simulink model "DSM_SIM"  (R2017b)
settings: Solver=FixedStepDiscrete  StartTime=0.0  StopTime=N/Fs  RelTol=1e-3
values from neighbouring files (symbols this model uses):
  ftest = 9e3    (= 9000)    [Model3.m]    (also in Model3_LTE.m = 2250)
  Ts = 1/Fs    (= 2.03450520833e-06)    [Model3.m]    (also in Model3_LTE.m = 1/Fs)
undefined symbols (not defined in the file or in its folder): a, b, c, g
libraries: dspsrcs4 x1
settings Model: Creator=o_cotte  LastModifiedBy=o_cotte

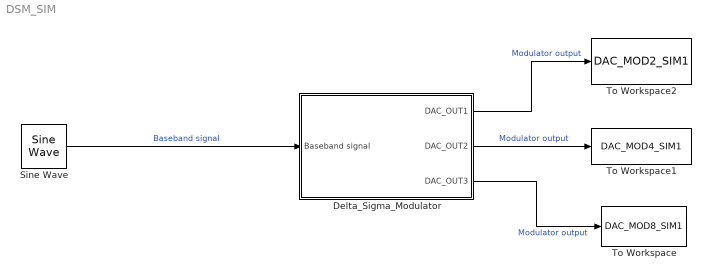
== system DSM_SIM ==
  Delta_Sigma_Modulator : Subsystem
  Sine Wave : dspsrcs4/Sine Wave  Amplitude=0.77  Frequency=ftest  Phase=0  SampleMode=Discrete  OutComplex=Real  CompMethod=Trigonometric fcn  TableSize=Speed  SampleTime=Ts  SamplesPerFrame=1  ResetState=Restart at time zero  OutputFrames=on  dataType=double  wordLen=16  udDataType=sfix(16)  fracBitsMode=Best precision  numFracBits=15  OutDataTypeStr=double  LastOutDataTypeStr=double
  To Workspace : ToWorkspace  VariableName=DAC_MOD8_SIM1  SampleTime=-1
  To Workspace1 : ToWorkspace  VariableName=DAC_MOD4_SIM1  SampleTime=-1
  To Workspace2 : ToWorkspace  VariableName=DAC_MOD2_SIM1  SampleTime=-1
  wires:
  Sine Wave/1 -> Delta_Sigma_Modulator/1(Baseband signal)  "Baseband signal"
  Delta_Sigma_Modulator/3(DAC_OUT3) -> To Workspace/1  "Modulator output"
  Delta_Sigma_Modulator/2(DAC_OUT2) -> To Workspace1/1  "Modulator output"
  Delta_Sigma_Modulator/1(DAC_OUT1) -> To Workspace2/1  "Modulator output"

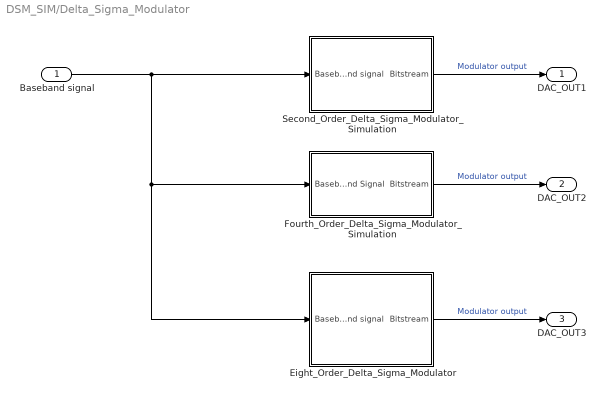
== system DSM_SIM/Delta_Sigma_Modulator ==
  Baseband signal : Inport
  Eight_Order_Delta_Sigma_Modulator : Subsystem
  Fourth_Order_Delta_Sigma_Modulator_Simulation : Subsystem
  Second_Order_Delta_Sigma_Modulator_Simulation : Subsystem
  DAC_OUT1 : Outport
  DAC_OUT2 : Outport  Port=2
  DAC_OUT3 : Outport  Port=3
  wires:
  Second_Order_Delta_Sigma_Modulator_Simulation/1(Bitstream) -> DAC_OUT1/1  "Modulator output"
  Fourth_Order_Delta_Sigma_Modulator_Simulation/1(Bitstream) -> DAC_OUT2/1  "Modulator output"
  Eight_Order_Delta_Sigma_Modulator/1(Bitstream) -> DAC_OUT3/1  "Modulator output"
  Baseband signal/1 -> Eight_Order_Delta_Sigma_Modulator/1(Baseband signal), Fourth_Order_Delta_Sigma_Modulator_Simulation/1(Baseband Signal), Second_Order_Delta_Sigma_Modulator_Simulation/1(Baseband signal)

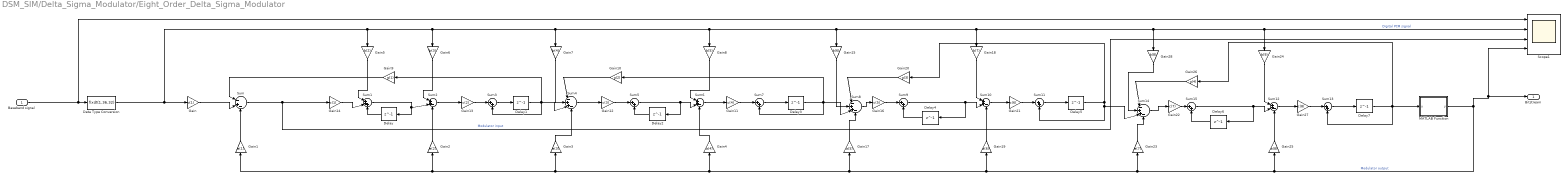
== system DSM_SIM/Delta_Sigma_Modulator/Eight_Order_Delta_Sigma_Modulator ==
  Baseband signal : Inport
  Data Type Conversion : DataTypeConversion  OutDataTypeStr=fixdt(1,36,32)
  Delay{,1..7} (8 alike) : Delay  DelayLength=1  InitialCondition=0
  Gain : Gain  Gain=b(1)  OutDataTypeStr=Inherit: Same as input  ParamDataTypeStr=Inherit: Same as input  LockScale=on
  Gain1 : Gain  Gain=a(1)  OutDataTypeStr=Inherit: Same as input
  Gain10 : Gain  Gain=g(2)  OutDataTypeStr=Inherit: Same as input  ParamDataTypeStr=Inherit: Same as input  LockScale=on
  Gain11 : Gain  Gain=c(4)  OutDataTypeStr=Inherit: Same as input  ParamDataTypeStr=Inherit: Same as input  LockScale=on
  Gain12 : Gain  Gain=c(3)  OutDataTypeStr=Inherit: Same as input  ParamDataTypeStr=Inherit: Same as input  LockScale=on
  Gain13 : Gain  Gain=c(2)  OutDataTypeStr=Inherit: Same as input  ParamDataTypeStr=Inherit: Same as input  LockScale=on
  Gain14 : Gain  Gain=c(1)  OutDataTypeStr=Inherit: Same as input  ParamDataTypeStr=Inherit: Same as input  LockScale=on
  Gain15 : Gain  Gain=b(6)  OutDataTypeStr=Inherit: Same as input  ParamDataTypeStr=Inherit: Same as input  LockScale=on
  Gain16 : Gain  Gain=c(5)  OutDataTypeStr=Inherit: Same as input  ParamDataTypeStr=Inherit: Same as input  LockScale=on
  Gain17 : Gain  Gain=a(5)  OutDataTypeStr=Inherit: Same as input
  Gain18 : Gain  Gain=b(7)  OutDataTypeStr=Inherit: Same as input  ParamDataTypeStr=Inherit: Same as input  LockScale=on
  Gain19 : Gain  Gain=a(6)  OutDataTypeStr=Inherit: Same as input
  Gain2 : Gain  Gain=a(2)  OutDataTypeStr=Inherit: Same as input
  Gain20 : Gain  Gain=g(3)  OutDataTypeStr=Inherit: Same as input  ParamDataTypeStr=Inherit: Same as input  LockScale=on
  Gain21 : Gain  Gain=c(6)  OutDataTypeStr=Inherit: Same as input  ParamDataTypeStr=Inherit: Same as input  LockScale=on
  Gain22 : Gain  Gain=c(7)  OutDataTypeStr=Inherit: Same as input  ParamDataTypeStr=Inherit: Same as input  LockScale=on
  Gain23 : Gain  Gain=a(7)  OutDataTypeStr=Inherit: Same as input
  Gain24 : Gain  Gain=b(9)  OutDataTypeStr=Inherit: Same as input  ParamDataTypeStr=Inherit: Same as input  LockScale=on
  Gain25 : Gain  Gain=a(8)  OutDataTypeStr=Inherit: Same as input
  Gain26 : Gain  Gain=g(4)  OutDataTypeStr=Inherit: Same as input  ParamDataTypeStr=Inherit: Same as input  LockScale=on
  Gain27 : Gain  Gain=c(8)  OutDataTypeStr=Inherit: Same as input  ParamDataTypeStr=Inherit: Same as input  LockScale=on
  Gain28 : Gain  Gain=b(8)  OutDataTypeStr=Inherit: Same as input  ParamDataTypeStr=Inherit: Same as input  LockScale=on
  Gain3 : Gain  Gain=a(3)  OutDataTypeStr=Inherit: Same as input
  Gain4 : Gain  Gain=a(4)  OutDataTypeStr=Inherit: Same as input
  Gain5 : Gain  Gain=b(2)  OutDataTypeStr=Inherit: Same as input  ParamDataTypeStr=Inherit: Same as input  LockScale=on
  Gain6 : Gain  Gain=b(3)  OutDataTypeStr=Inherit: Same as input  ParamDataTypeStr=Inherit: Same as input  LockScale=on
  Gain7 : Gain  Gain=b(4)  OutDataTypeStr=Inherit: Same as input  ParamDataTypeStr=Inherit: Same as input  LockScale=on
  Gain8 : Gain  Gain=b(5)  OutDataTypeStr=Inherit: Same as input  ParamDataTypeStr=Inherit: Same as input  LockScale=on
  Gain9 : Gain  Gain=g(1)  OutDataTypeStr=Inherit: Same as input  ParamDataTypeStr=Inherit: Same as input  LockScale=on
  MATLAB Function : MATLAB Function  TreatAsAtomicUnit=on
  Scope1 : Scope  NumInputPorts=4
  Sum : Sum  Inputs=|-+-  OutDataTypeStr=Inherit: Same as accumulator  LockScale=on
  Sum1 : Sum  Inputs=|+++  OutDataTypeStr=Inherit: Same as accumulator  LockScale=on
  Sum{2,6,10,12} (4 alike) : Sum  Inputs=|++-  OutDataTypeStr=Inherit: Same as accumulator  LockScale=on
  Sum{3,5,7,9,11,13,15} (7 alike) : Sum  Inputs=|++  OutDataTypeStr=Inherit: Same as accumulator  LockScale=on
  Sum14 : Sum  Inputs=|-++-  OutDataTypeStr=Inherit: Same as accumulator  LockScale=on
  Sum4 : Sum  Inputs=|-++-  OutDataTypeStr=Inherit: Same as accumulator  LockScale=on
  Sum8 : Sum  Inputs=|-++-  OutDataTypeStr=Inherit: Same as accumulator  LockScale=on
  Bitstream : Outport
  wires:
  Delay5/1 -> Sum14/3, Sum11/2, Gain20/1
  Gain27/1 -> Sum13/1
  Gain26/1 -> Sum14/1
  Gain16/1 -> Sum9/1
  Gain13/1 -> Sum3/1
  Gain6/1 -> Sum2/1
  Delay7/1 -> MATLAB Function/1(u), Sum13/2, Gain26/1
  Gain7/1 -> Sum4/2
  Gain23/1 -> Sum14/4
  Gain28/1 -> Sum14/2
  Gain19/1 -> Sum10/3
  Gain24/1 -> Sum12/1
  Delay4/1 -> Sum9/2
  Gain15/1 -> Sum8/2
  Sum15/1 -> Delay6/1, Sum12/2
  Gain22/1 -> Sum15/1
  Gain25/1 -> Sum12/3
  Sum13/1 -> Delay7/1
  Sum14/1 -> Gain22/1
  Gain18/1 -> Sum10/1
  MATLAB Function/1(y) -> Bitstream/1, Scope1/4, Gain25/1, Gain23/1, Gain19/1, Gain17/1, Gain1/1, Gain2/1, Gain3/1, Gain4/1  "Modulator output"
  Sum8/1 -> Gain16/1
  Delay6/1 -> Sum15/2
  Sum5/1 -> Delay2/1, Sum6/2
  Baseband signal/1 -> Data Type Conversion/1, Scope1/1
  Gain14/1 -> Sum1/2
  Sum6/1 -> Gain11/1
  Data Type Conversion/1 -> Gain5/1, Gain8/1, Gain18/1, Gain28/1, Gain24/1, Scope1/2, Gain15/1, Gain7/1, Gain6/1, Gain/1  "Digital PCM signal"
  Sum12/1 -> Gain27/1
  Sum/1 -> Scope1/3, Gain14/1  "Modulator input"
  Delay2/1 -> Sum5/2
  Delay1/1 -> Sum3/2, Gain9/1, Sum4/3
  Sum9/1 -> Delay4/1, Sum10/2
  Sum4/1 -> Gain12/1
  Sum11/1 -> Delay5/1
  Sum2/1 -> Gain13/1
  Gain20/1 -> Sum8/1
  Sum7/1 -> Delay3/1
  Gain5/1 -> Sum1/1
  Gain8/1 -> Sum6/1
  Gain10/1 -> Sum4/1
  Gain11/1 -> Sum7/1
  Gain21/1 -> Sum11/1
  Gain/1 -> Sum/2
  Sum1/1 -> Delay/1, Sum2/2
  Gain12/1 -> Sum5/1
  Gain9/1 -> Sum/1
  Gain4/1 -> Sum6/3
  Gain17/1 -> Sum8/4
  Sum10/1 -> Gain21/1
  Delay3/1 -> Sum8/3, Sum7/2, Gain10/1
  Gain2/1 -> Sum2/3
  Gain3/1 -> Sum4/4
  Gain1/1 -> Sum/3
  Delay/1 -> Sum1/3
  Sum3/1 -> Delay1/1

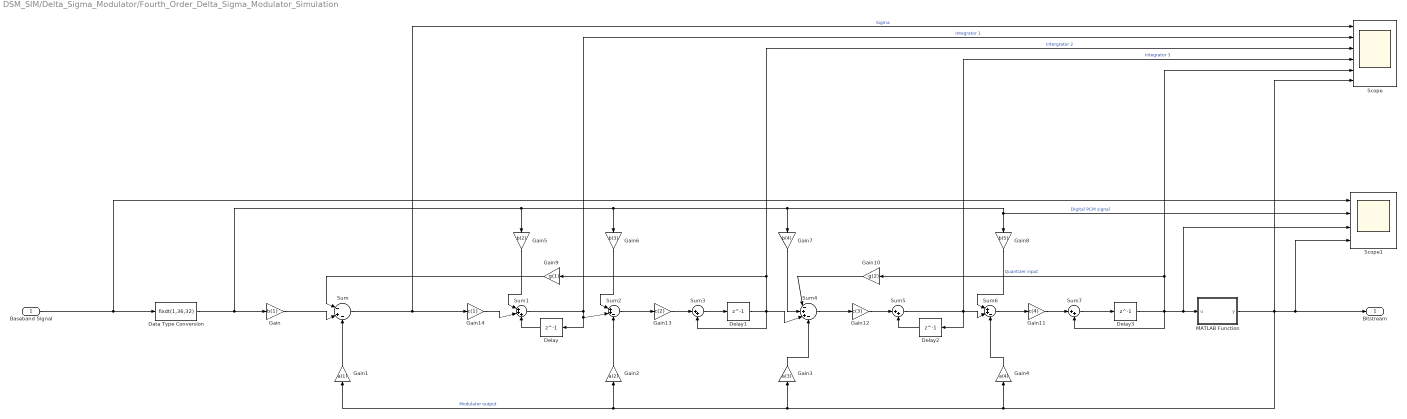
== system DSM_SIM/Delta_Sigma_Modulator/Fourth_Order_Delta_Sigma_Modulator_Simulation ==
  Baseband Signal : Inport
  Data Type Conversion : DataTypeConversion  OutDataTypeStr=fixdt(1,36,32)
  Delay{,1..3} (4 alike) : Delay  DelayLength=1  InitialCondition=0
  Gain : Gain  Gain=b(1)  OutDataTypeStr=Inherit: Same as input  ParamDataTypeStr=Inherit: Same as input  LockScale=on
  Gain1 : Gain  Gain=a(1)  OutDataTypeStr=Inherit: Same as input
  Gain10 : Gain  Gain=g(2)  OutDataTypeStr=Inherit: Same as input  ParamDataTypeStr=Inherit: Same as input  LockScale=on
  Gain11 : Gain  Gain=c(4)  OutDataTypeStr=Inherit: Same as input  ParamDataTypeStr=Inherit: Same as input  LockScale=on
  Gain12 : Gain  Gain=c(3)  OutDataTypeStr=Inherit: Same as input  ParamDataTypeStr=Inherit: Same as input  LockScale=on
  Gain13 : Gain  Gain=c(2)  OutDataTypeStr=Inherit: Same as input  ParamDataTypeStr=Inherit: Same as input  LockScale=on
  Gain14 : Gain  Gain=c(1)  OutDataTypeStr=Inherit: Same as input  ParamDataTypeStr=Inherit: Same as input  LockScale=on
  Gain2 : Gain  Gain=a(2)  OutDataTypeStr=Inherit: Same as input
  Gain3 : Gain  Gain=a(3)  OutDataTypeStr=Inherit: Same as input
  Gain4 : Gain  Gain=a(4)  OutDataTypeStr=Inherit: Same as input
  Gain5 : Gain  Gain=b(2)  OutDataTypeStr=Inherit: Same as input  ParamDataTypeStr=Inherit: Same as input  LockScale=on
  Gain6 : Gain  Gain=b(3)  OutDataTypeStr=Inherit: Same as input  ParamDataTypeStr=Inherit: Same as input  LockScale=on
  Gain7 : Gain  Gain=b(4)  OutDataTypeStr=Inherit: Same as input  ParamDataTypeStr=Inherit: Same as input  LockScale=on
  Gain8 : Gain  Gain=b(5)  OutDataTypeStr=Inherit: Same as input  ParamDataTypeStr=Inherit: Same as input  LockScale=on
  Gain9 : Gain  Gain=g(1)  OutDataTypeStr=Inherit: Same as input  ParamDataTypeStr=Inherit: Same as input  LockScale=on
  MATLAB Function : MATLAB Function  TreatAsAtomicUnit=on
  Scope : Scope  NumInputPorts=6
  Scope1 : Scope  NumInputPorts=4
  Sum : Sum  Inputs=|-+-  OutDataTypeStr=Inherit: Same as accumulator  LockScale=on
  Sum1 : Sum  Inputs=|+++  OutDataTypeStr=Inherit: Same as accumulator  LockScale=on
  Sum2 : Sum  Inputs=|++-  OutDataTypeStr=Inherit: Same as accumulator  LockScale=on
  Sum3 : Sum  Inputs=|++  OutDataTypeStr=Inherit: Same as accumulator  LockScale=on
  Sum4 : Sum  Inputs=|-++-  OutDataTypeStr=Inherit: Same as accumulator  LockScale=on
  Sum5 : Sum  Inputs=|++  OutDataTypeStr=Inherit: Same as accumulator  LockScale=on
  Sum6 : Sum  Inputs=|++-  OutDataTypeStr=Inherit: Same as accumulator  LockScale=on
  Sum7 : Sum  Inputs=|++  OutDataTypeStr=Inherit: Same as accumulator  LockScale=on
  Bitstream : Outport
  wires:
  Sum1/1 -> Scope/2, Delay/1, Sum2/2  "Integrator 1"
  Sum3/1 -> Delay1/1
  Gain5/1 -> Sum1/1
  Delay3/1 -> Scope1/3, MATLAB Function/1(u), Sum7/2, Scope/5, Gain10/1  "Quantizer input"
  MATLAB Function/1(y) -> Scope/6, Bitstream/1, Scope1/4, Gain1/1, Gain2/1, Gain3/1, Gain4/1  "Modulator output"
  Sum4/1 -> Gain12/1
  Gain11/1 -> Sum7/1
  Sum2/1 -> Gain13/1
  Gain6/1 -> Sum2/1
  Gain7/1 -> Sum4/2
  Gain10/1 -> Sum4/1
  Gain13/1 -> Sum3/1
  Sum5/1 -> Scope/4, Delay2/1, Sum6/2  "Integrator 3"
  Gain/1 -> Sum/2
  Baseband Signal/1 -> Data Type Conversion/1, Scope1/1
  Delay2/1 -> Sum5/2
  Data Type Conversion/1 -> Gain5/1, Gain8/1, Scope1/2, Gain7/1, Gain6/1, Gain/1  "Digital PCM signal"
  Sum6/1 -> Gain11/1
  Gain2/1 -> Sum2/3
  Gain8/1 -> Sum6/1
  Gain14/1 -> Sum1/2
  Gain3/1 -> Sum4/4
  Gain4/1 -> Sum6/3
  Delay/1 -> Sum1/3
  Sum7/1 -> Delay3/1
  Gain12/1 -> Sum5/1
  Gain1/1 -> Sum/3
  Gain9/1 -> Sum/1
  Sum/1 -> Scope/1, Gain14/1  "Sigma"
  Delay1/1 -> Sum3/2, Scope/3, Gain9/1, Sum4/3  "Intergrator 2"

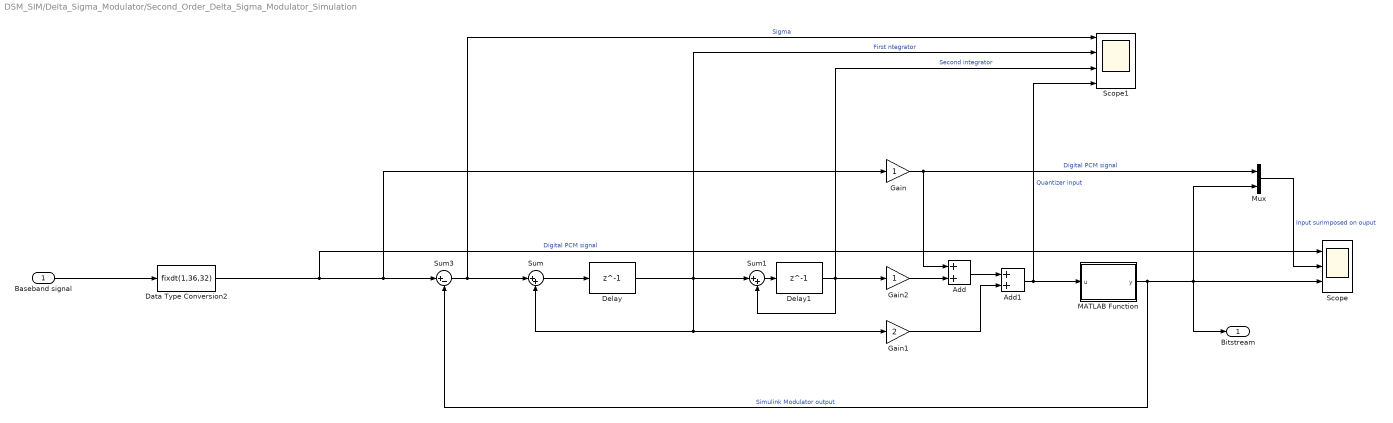
== system DSM_SIM/Delta_Sigma_Modulator/Second_Order_Delta_Sigma_Modulator_Simulation ==
  Baseband signal : Inport
  Add : Sum  OutDataTypeStr=Inherit: Same as accumulator  LockScale=on
  Add1 : Sum  OutDataTypeStr=Inherit: Same as accumulator
  Data Type Conversion2 : DataTypeConversion  OutDataTypeStr=fixdt(1,36,32)  LockScale=on
  Delay : Delay  DelayLength=1  InitialCondition=0  InputProcessing=Columns as channels (frame based)
  Delay1 : Delay  DelayLength=1  InitialCondition=0  InputProcessing=Columns as channels (frame based)
  Gain : Gain  OutDataTypeStr=Inherit: Same as input  LockScale=on
  Gain1 : Gain  Gain=2  OutDataTypeStr=Inherit: Same as input  ParamDataTypeStr=Inherit: Same as input  LockScale=on
  Gain2 : Gain  OutDataTypeStr=Inherit: Same as input  LockScale=on
  MATLAB Function : MATLAB Function  TreatAsAtomicUnit=on
  Mux : Mux  Inputs=2
  Scope : Scope  NumInputPorts=3
  Scope1 : Scope  NumInputPorts=4
  Sum : Sum  Inputs=|++  OutDataTypeStr=Inherit: Same as accumulator
  Sum1 : Sum  Inputs=|++  OutDataTypeStr=Inherit: Same as accumulator
  Sum3 : Sum  Inputs=|+-  OutDataTypeStr=Inherit: Same as accumulator
  Bitstream : Outport
  wires:
  Mux/1 -> Scope/2  "Input surimposed on ouput"
  Gain2/1 -> Add/2
  Sum/1 -> Delay/1
  Gain1/1 -> Add1/2
  Delay1/1 -> Gain2/1, Scope1/3, Sum1/2  "Second integrator"
  Sum1/1 -> Delay1/1
  MATLAB Function/1(y) -> Sum3/2, Bitstream/1, Mux/2, Scope/3  "Simulink Modulator output"
  Delay/1 -> Scope1/2, Sum1/1, Gain1/1, Sum/2  "First ntegrator"
  Gain/1 -> Add/1, Mux/1  "Digital PCM signal"
  Sum3/1 -> Sum/1, Scope1/1  "Sigma"
  Data Type Conversion2/1 -> Gain/1, Sum3/1, Scope/1  "Digital PCM signal"
  Add/1 -> Add1/1
  Baseband signal/1 -> Data Type Conversion2/1
  Add1/1 -> MATLAB Function/1(u), Scope1/4  "Quantizer input"

== matlab function DSM_SIM/Delta_Sigma_Modulator/Second_Order_Delta_Sigma_Modulator_Simulation/MATLAB Function ==
  data: u input; y output
function y = fcn(u)
%#codegen
% nLev=2;
% st=fi(nLev-2,1,36,30);
% y=fi(0,1,36,30);
% if u < -st
%     y = fi(-nLev+1,1,36,30);
% elseif u >= st
%     y = fi(nLev-1,1,36,30);
% else
%     for n=1:nLev-2
%         k=fi(n,1,36,30);
%         if u >= -nLev + 2*k && u < -nLev + 2*(k+1)
%             y = fi(2*k-1-nLev,1,36,30);
%         end
%     end
% end
% nLev=64;
% st=fi(nLev-2,1,36,25);
% y=fi(0,1,36,25);
% for n=1:nLev-2
%     k=fi(n,1,36,25);
%     if u < -st
%         y = fi(-nLev+1,1,36,25);
%         break;
%     elseif u >= st
%         y = fi(nLev-1,1,36,25);
%         break;
%     elseif u >= -nLev + 2*k && u < -nLev + 2*(k+1)
%         y = fi(2*k-1-nLev,1,36,25);
%         break;
%     end
% end

if u < 0
    y = fi(-1,1,36,32);
    %y = -1;
else
    y = fi(1,1,36,32);
    %y = 1;
end

% if u < -14
%     y = fi(-15,1,36,28);
% elseif u >= -14 && u < -12
%     y = fi(-13,1,36,28);
% elseif u >= -12 && u < -10
%     y = fi(-11,1,36,28);
% elseif u >= -10 && u < -8
%     y = fi(-9,1,36,28);
% elseif u >= -8 && u < -6
%     y = fi(-7,1,36,28);
% elseif u >= -6 && u < -4
%     y = fi(-5,1,36,28);
% elseif u >= -4 && u < -2
%     y = fi(-3,1,36,28);
% elseif u >= -2 && u < 0
%     y = fi(-1,1,36,28);
% elseif u >= 0 && u < 2
%     y = fi(1,1,36,28);
% elseif u >= 2 && u < 4
%     y = fi(3,1,36,28);
% elseif u >= 4 && u < 6
%     y = fi(5,1,36,28);
% elseif u >= 6 && u < 8
%     y = fi(7,1,36,28);
% elseif u >= 8 && u < 10
%     y = fi(9,1,36,28);
% elseif u >= 10 && u < 12
%     y = fi(11,1,36,28);
% elseif u >= 12 && u < 14
%     y = fi(13,1,36,28);
% else % u > 14
%     y = fi(15,1,36,28);
% end

== matlab function DSM_SIM/Delta_Sigma_Modulator/Fourth_Order_Delta_Sigma_Modulator_Simulation/MATLAB Function ==
  data: u input; y output
function y = fcn(u)
%#codegen
% nLev=64;
% st=fi(nLev-2,1,36,28);
% y=fi(1,1,36,28);
% for n=1:nLev-2
%     k=fi(n,1,36,28);
%     if u < -st
%         y=fi(-nLev+1,1,36,28);
%         break;
%     elseif u > st
%         y=fi(nLev-1,1,36,28);
%         break;
%     elseif u >= -nLev + 2*k && u <= -nLev + 2*(k+1)
%         y=fi(2*k-1-nLev,1,36,28);
%         break;
%     end
% end

% 2-level
if u < 0
    y = fi(-1,1,36,32);
    %y = -1;
else
    y = fi(1,1,36,32);
    %y = 1;
end

% 4-level
% if u < -2
%     y = fi(-3,1,36,28);
% elseif u > -2 && u < 0
%     y = fi(-1,1,36,28);
% elseif u >= 0 && u < 2
%     y = fi(1,1,36,28);
% else
%     y = fi(3,1,36,28);
% end

% 64-level
% if u < -62
%     y = fi(-63,1,36,28);
% elseif u >= -62 && u < -60
%     y = fi(-61,1,36,28);
% elseif u >= -60 && u < -58
%     y = fi(-59,1,36,28);
% elseif u >= -58 && u < -56
%     y = fi(-57,1,36,28);
% elseif u >= -56 && u < -54
%     y = fi(-55,1,36,28);
% elseif u >= -54 && u < -52
%     y = fi(-53,1,36,28);
% elseif u >= -52 && u < -50
%     y = fi(-51,1,36,28);
% elseif u >= -50 && u < -48
%     y = fi(-49,1,36,28);
% elseif u >= -48 && u < -46
%     y = fi(-47,1,36,28);
% elseif u >= -46 && u < -44
%     y = fi(-45,1,36,28);
% elseif u >= -44 && u < -42
%     y = fi(-43,1,36,28);
% elseif u >= -42 && u < -40
%     y = fi(-41,1,36,28);
% elseif u >= -40 && u < -38
%     y = fi(-39,1,36,28);
% elseif u >= -38 && u < -36
%     y = fi(-37,1,36,28);
% elseif u >= -36 && u < -34
%     y = fi(-35,1,36,28);
% elseif u >= -34 && u < -32
%     y = fi(-33,1,36,28);
% elseif u >= -32 && u < -30
%     y = fi(-31,1,36,28);
% elseif u >= -30 && u < -28
%     y = fi(-29,1,36,28);
% elseif u >= -28 && u < -26
%     y = fi(-27,1,36,28);
% elseif u >= -26 && u < -24
%     y = fi(-25,1,36,28);
% elseif u >= -24 && u < -22
%     y = fi(-23,1,36,28);
% elseif u >= -22 && u < -20
%     y = fi(-21,1,36,28);
% elseif u >= -20 && u < -18
%     y = fi(-19,1,36,28);
% elseif u >= -18 && u < -16
%     y = fi(-17,1,36,28);
% elseif u >= -16 && u < -14
%     y = fi(-15,1,36,28);
% elseif u >= -14 && u < -12
%     y = fi(-13,1,36,28);
% elseif u >= -12 && u < -10
%     y = fi(-11,1,36,28);
% elseif u >= -10 && u < -8
%     y = fi(-9,1,36,28);
% elseif u >= -8 && u < -6
%     y = fi(-7,1,36,28);
% elseif u >= -6 && u < -4
%     y = fi(-5,1,36,28);
% elseif u >= -4 && u < -2
%     y = fi(-3,1,36,28);
% elseif u >= -2 && u < 0
%     y = fi(-1,1,36,28);
% elseif u >= 0 && u < 2
%     y = fi(1,1,36,28);
% elseif u >= 2 && u < 4
%     y = fi(3,1,36,28);
% elseif u >= 4 && u < 6
%     y = fi(5,1,36,28);
% elseif u >= 6 && u < 8
%     y = fi(7,1,36,28);
% elseif u >= 8 && u < 10
%     y = fi(9,1,36,28);
% elseif u >= 10 && u < 12
%     y = fi(11,1,36,28);
% elseif u >= 12 && u < 14
%     y = fi(13,1,36,28);
% elseif u >= 14 && u < 16
%     y = fi(15,1,36,28);
% elseif u >= 16 && u < 18
%     y = fi(17,1,36,28);
% elseif u >= 18 && u < 20
%     y = fi(19,1,36,28);
% elseif u >= 20 && u < 22
%     y = fi(21,1,36,28);
% elseif u >= 22 && u < 24
%     y = fi(23,1,36,28);
% elseif u >= 24 && u < 26
%     y = fi(25,1,36,28);
% elseif u >= 26 && u < 28
%     y = fi(27,1,36,28);
% elseif u >= 28 && u < 30
%     y = fi(29,1,36,28);
% elseif u >= 30 && u < 32
%     y = fi(31,1,36,28);
% elseif u >= 32 && u < 34
%     y = fi(33,1,36,28);
% elseif u >= 34 && u < 36
%     y = fi(35,1,36,28);
% elseif u >= 36 && u < 38
%     y = fi(37,1,36,28);
% elseif u >= 38 && u < 40
%     y = fi(39,1,36,28);
% elseif u >= 40 && u < 42
%     y = fi(41,1,36,28);
% elseif u >= 42 && u < 44
%     y = fi(43,1,36,28);
% elseif u >= 44 && u < 46
%     y = fi(45,1,36,28);
% elseif u >= 46 && u < 48
%     y = fi(47,1,36,28);
% elseif u >= 48 && u < 50
%     y = fi(49,1,36,28);
% elseif u >= 50 && u < 52
%     y = fi(51,1,36,28);
% elseif u >= 52 && u < 54
%     y = fi(53,1,36,28);
% elseif u >= 54 && u < 56
%     y = fi(55,1,36,28);
% elseif u >= 56 && u < 58
%     y = fi(57,1,36,28);
% elseif u >= 58 && u < 60
%     y = fi(59,1,36,28);
% elseif u >= 60 && u < 62
%     y = fi(61,1,36,28);
% else % u > 62
%     y = fi(63,1,36,28);
% end

% 32-level
% if u < -30
%     y = fi(-31,1,36,28);
% elseif u >= -30 && u < -28
%     y = fi(-29,1,36,28);
% elseif u >= -28 && u < -26
%     y = fi(-27,1,36,28);
% elseif u >= -26 && u < -24
%     y = fi(-25,1,36,28);
% elseif u >= -24 && u < -22
%     y = fi(-23,1,36,28);
% elseif u >= -22 && u < -20
%     y = fi(-21,1,36,28);
% elseif u >= -20 && u < -18
%     y = fi(-19,1,36,28);
% elseif u >= -18 && u < -16
%     y = fi(-17,1,36,28);
% elseif u >= -16 && u < -14
%     y = fi(-15,1,36,28);
% elseif u >= -14 && u < -12
%     y = fi(-13,1,36,28);
% elseif u >= -12 && u < -10
%     y = fi(-11,1,36,28);
% elseif u >= -10 && u < -8
%     y = fi(-9,1,36,28);
% elseif u >= -8 && u < -6
%     y = fi(-7,1,36,28);
% elseif u >= -6 && u < -4
%     y = fi(-5,1,36,28);
% elseif u >= -4 && u < -2
%     y = fi(-3,1,36,28);
% elseif u >= -2 && u < 0
%     y = fi(-1,1,36,28);
% elseif u >= 0 && u < 2
%     y = fi(1,1,36,28);
% elseif u >= 2 && u < 4
%     y = fi(3,1,36,28);
% elseif u >= 4 && u < 6
%     y = fi(5,1,36,28);
% elseif u >= 6 && u < 8
%     y = fi(7,1,36,28);
% elseif u >= 8 && u < 10
%     y = fi(9,1,36,28);
% elseif u >= 10 && u < 12
%     y = fi(11,1,36,28);
% elseif u >= 12 && u < 14
%     y = fi(13,1,36,28);
% elseif u >= 14 && u < 16
%     y = fi(15,1,36,28);
% elseif u >= 16 && u < 18
%     y = fi(17,1,36,28);
% elseif u >= 18 && u < 20
%     y = fi(19,1,36,28);
% elseif u >= 20 && u < 22
%     y = fi(21,1,36,28);
% elseif u >= 22 && u < 24
%     y = fi(23,1,36,28);
% elseif u >= 24 && u < 26
%     y = fi(25,1,36,28);
% elseif u >= 26 && u < 28
%     y = fi(27,1,36,28);
% elseif u >= 28 && u < 30
%     y = fi(29,1,36,28);
% else % u > 30
%     y = fi(31,1,36,28);
% end

== matlab function DSM_SIM/Delta_Sigma_Modulator/Eight_Order_Delta_Sigma_Modulator/MATLAB Function ==
  data: u input; y output
function y = fcn(u)
%#codegen
% nLev=32;
% st=fi(nLev-2,1,36,28);
% y=fi(1,1,36,28);
% for n=1:nLev-2
%     k=fi(n,1,36,28);
%     if u < -st
%         y=fi(-nLev+1,1,36,28);
%         break;
%     elseif u > st
%         y=fi(nLev-1,1,36,28);
%         break;
%     elseif u >= -nLev + 2*k && u <= -nLev + 2*(k+1)
%         y=fi(2*k-1-nLev,1,36,28);
%         break;
%     end
% end
% nLev=2;
% st=fi(nLev,1,36,28);
% y=fi(0,1,36,28);
% for n=1:nLev
%     k=fi(n,1,36,28);
%     if u < -st+2
%         y = fi(-nLev+1,1,36,28);
%         break;
%     elseif u < -nLev + 2*k && u > -nLev + 2*(k+1)
%         y = fi(-nLev+1,1,36,28);
%         break;
%     elseif u >= nLev - 2*k && u < nLev - 2*(k+1)
%         y = fi(-nLev+1,1,36,28);
%         break;
%     else u > st-2
%         y = fi(nLev-1,1,36,28);
%         break;
%     end
% end

% 2-level
% if u < 0
%     y = -1;
% else
%     y = 1;
% end

% 2-level
if u < 0
    y = fi(-1,1,36,32);
else
    y = fi(1,1,36,32);
end

% 4-level
% if u < -2
%     y = fi(-3,1,36,28);
% elseif u > -2 && u < 0
%     y = fi(-1,1,36,28);
% elseif u >= 0 && u < 2
%     y = fi(1,1,36,28);
% else
%     y = fi(3,1,36,28);
% end

% 64-level
% if u < -62
%     y = fi(-63,1,36,28);
% elseif u >= -62 && u < -60
%     y = fi(-61,1,36,28);
% elseif u >= -60 && u < -58
%     y = fi(-59,1,36,28);
% elseif u >= -58 && u < -56
%     y = fi(-57,1,36,28);
% elseif u >= -56 && u < -54
%     y = fi(-55,1,36,28);
% elseif u >= -54 && u < -52
%     y = fi(-53,1,36,28);
% elseif u >= -52 && u < -50
%     y = fi(-51,1,36,28);
% elseif u >= -50 && u < -48
%     y = fi(-49,1,36,28);
% elseif u >= -48 && u < -46
%     y = fi(-47,1,36,28);
% elseif u >= -46 && u < -44
%     y = fi(-45,1,36,28);
% elseif u >= -44 && u < -42
%     y = fi(-43,1,36,28);
% elseif u >= -42 && u < -40
%     y = fi(-41,1,36,28);
% elseif u >= -40 && u < -38
%     y = fi(-39,1,36,28);
% elseif u >= -38 && u < -36
%     y = fi(-37,1,36,28);
% elseif u >= -36 && u < -34
%     y = fi(-35,1,36,28);
% elseif u >= -34 && u < -32
%     y = fi(-33,1,36,28);
% elseif u >= -32 && u < -30
%     y = fi(-31,1,36,28);
% elseif u >= -30 && u < -28
%     y = fi(-29,1,36,28);
% elseif u >= -28 && u < -26
%     y = fi(-27,1,36,28);
% elseif u >= -26 && u < -24
%     y = fi(-25,1,36,28);
% elseif u >= -24 && u < -22
%     y = fi(-23,1,36,28);
% elseif u >= -22 && u < -20
%     y = fi(-21,1,36,28);
% elseif u >= -20 && u < -18
%     y = fi(-19,1,36,28);
% elseif u >= -18 && u < -16
%     y = fi(-17,1,36,28);
% elseif u >= -16 && u < -14
%     y = fi(-15,1,36,28);
% elseif u >= -14 && u < -12
%     y = fi(-13,1,36,28);
% elseif u >= -12 && u < -10
%     y = fi(-11,1,36,28);
% elseif u >= -10 && u < -8
%     y = fi(-9,1,36,28);
% elseif u >= -8 && u < -6
%     y = fi(-7,1,36,28);
% elseif u >= -6 && u < -4
%     y = fi(-5,1,36,28);
% elseif u >= -4 && u < -2
%     y = fi(-3,1,36,28);
% elseif u >= -2 && u < 0
%     y = fi(-1,1,36,28);
% elseif u >= 0 && u < 2
%     y = fi(1,1,36,28);
% elseif u >= 2 && u < 4
%     y = fi(3,1,36,28);
% elseif u >= 4 && u < 6
%     y = fi(5,1,36,28);
% elseif u >= 6 && u < 8
%     y = fi(7,1,36,28);
% elseif u >= 8 && u < 10
%     y = fi(9,1,36,28);
% elseif u >= 10 && u < 12
%     y = fi(11,1,36,28);
% elseif u >= 12 && u < 14
%     y = fi(13,1,36,28);
% elseif u >= 14 && u < 16
%     y = fi(15,1,36,28);
% elseif u >= 16 && u < 18
%     y = fi(17,1,36,28);
% elseif u >= 18 && u < 20
%     y = fi(19,1,36,28);
% elseif u >= 20 && u < 22
%     y = fi(21,1,36,28);
% elseif u >= 22 && u < 24
%     y = fi(23,1,36,28);
% elseif u >= 24 && u < 26
%     y = fi(25,1,36,28);
% elseif u >= 26 && u < 28
%     y = fi(27,1,36,28);
% elseif u >= 28 && u < 30
%     y = fi(29,1,36,28);
% elseif u >= 30 && u < 32
%     y = fi(31,1,36,28);
% elseif u >= 32 && u < 34
%     y = fi(33,1,36,28);
% elseif u >= 34 && u < 36
%     y = fi(35,1,36,28);
% elseif u >= 36 && u < 38
%     y = fi(37,1,36,28);
% elseif u >= 38 && u < 40
%     y = fi(39,1,36,28);
% elseif u >= 40 && u < 42
%     y = fi(41,1,36,28);
% elseif u >= 42 && u < 44
%     y = fi(43,1,36,28);
% elseif u >= 44 && u < 46
%     y = fi(45,1,36,28);
% elseif u >= 46 && u < 48
%     y = fi(47,1,36,28);
% elseif u >= 48 && u < 50
%     y = fi(49,1,36,28);
% elseif u >= 50 && u < 52
%     y = fi(51,1,36,28);
% elseif u >= 52 && u < 54
%     y = fi(53,1,36,28);
% elseif u >= 54 && u < 56
%     y = fi(55,1,36,28);
% elseif u >= 56 && u < 58
%     y = fi(57,1,36,28);
% elseif u >= 58 && u < 60
%     y = fi(59,1,36,28);
% elseif u >= 60 && u < 62
%     y = fi(61,1,36,28);
% else % u > 62
%     y = fi(63,1,36,28);
% end

% 32-level
% if u < -30
%     y = fi(-31,1,36,28);
% elseif u >= -30 && u < -28
%     y = fi(-29,1,36,28);
% elseif u >= -28 && u < -26
%     y = fi(-27,1,36,28);
% elseif u >= -26 && u < -24
%     y = fi(-25,1,36,28);
% elseif u >= -24 && u < -22
%     y = fi(-23,1,36,28);
% elseif u >= -22 && u < -20
%     y = fi(-21,1,36,28);
% elseif u >= -20 && u < -18
%     y = fi(-19,1,36,28);
% elseif u >= -18 && u < -16
%     y = fi(-17,1,36,28);
% elseif u >= -16 && u < -14
%     y = fi(-15,1,36,28);
% elseif u >= -14 && u < -12
%     y = fi(-13,1,36,28);
% elseif u >= -12 && u < -10
%     y = fi(-11,1,36,28);
% elseif u >= -10 && u < -8
%     y = fi(-9,1,36,28);
% elseif u >= -8 && u < -6
%     y = fi(-7,1,36,28);
% elseif u >= -6 && u < -4
%     y = fi(-5,1,36,28);
% elseif u >= -4 && u < -2
%     y = fi(-3,1,36,28);
% elseif u >= -2 && u < 0
%     y = fi(-1,1,36,28);
% elseif u >= 0 && u < 2
%     y = fi(1,1,36,28);
% elseif u >= 2 && u < 4
%     y = fi(3,1,36,28);
% elseif u >= 4 && u < 6
%     y = fi(5,1,36,28);
% elseif u >= 6 && u < 8
%     y = fi(7,1,36,28);
% elseif u >= 8 && u < 10
%     y = fi(9,1,36,28);
% elseif u >= 10 && u < 12
%     y = fi(11,1,36,28);
% elseif u >= 12 && u < 14
%     y = fi(13,1,36,28);
% elseif u >= 14 && u < 16
%     y = fi(15,1,36,28);
% elseif u >= 16 && u < 18
%     y = fi(17,1,36,28);
% elseif u >= 18 && u < 20
%     y = fi(19,1,36,28);
% elseif u >= 20 && u < 22
%     y = fi(21,1,36,28);
% elseif u >= 22 && u < 24
%     y = fi(23,1,36,28);
% elseif u >= 24 && u < 26
%     y = fi(25,1,36,28);
% elseif u >= 26 && u < 28
%     y = fi(27,1,36,28);
% elseif u >= 28 && u < 30
%     y = fi(29,1,36,28);
% else % u > 30
%     y = fi(31,1,36,28);
% end
